simulink model "stateSpace"  (R2018a)
settings: Solver=VariableStepAuto  StartTime=0.0  StopTime=10.0  RelTol=1e-3
values from neighbouring files (symbols this model uses):
  K = place(Anew,Bnew,p)    [trackingControlScript.m]
undefined symbols (not defined in the file or in its folder): L
settings Model: Creator=Haydar  LastModifiedBy=Haydar

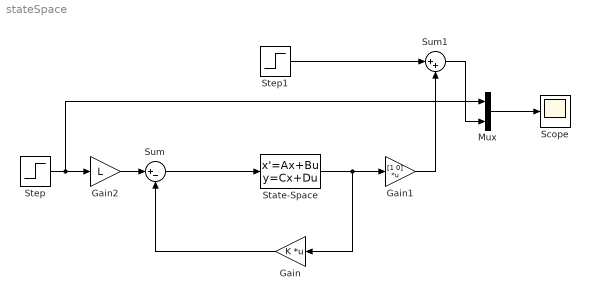
== system stateSpace ==
  Gain : Gain  Gain=K  Multiplication=Matrix(K*u)
  Gain1 : Gain  Gain=[1 0]  Multiplication=Matrix(K*u)
  Gain2 : Gain  Gain=L
  Mux : Mux  Inputs=2
  Scope : Scope
  State-Space : StateSpace  A=[-1 3;0 -2]  B=[1;1]  C=[1 0;0 1]  D=[0;0]  InitialCondition=0
  Step : Step  Time=0  SampleTime=0
  Step1 : Step  Time=5  SampleTime=0
  Sum : Sum  Inputs=|+-
  Sum1 : Sum  Inputs=|++
  wires:
  State-Space/1 -> Gain1/1, Gain/1
  Sum/1 -> State-Space/1
  Gain/1 -> Sum/2
  Step/1 -> Gain2/1, Mux/1
  Mux/1 -> Scope/1
  Gain2/1 -> Sum/1
  Step1/1 -> Sum1/1
  Gain1/1 -> Sum1/2
  Sum1/1 -> Mux/2
